simulink model "simulin"  (R2025b)
settings: Solver=VariableStepAuto  StartTime=0.0  StopTime=10.0  RelTol=1e-3
settings Model: Creator=viktor  LastModifiedBy=viktor

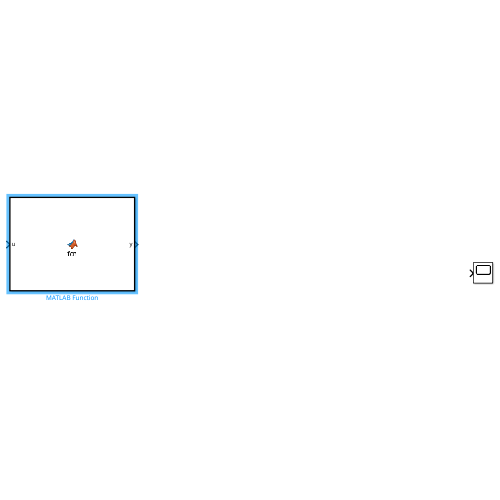
[thumbnail: Simulink's stored preview of the top-level diagram]
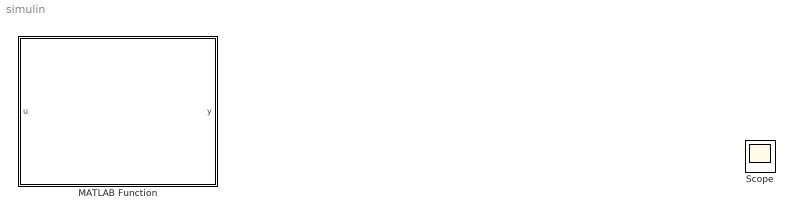
== system simulin ==
  MATLAB Function : MATLAB Function  TreatAsAtomicUnit=on
  Scope : Scope

== matlab function simulin/MATLAB Function ==
  data: u input; y output
function y = fcn(u)

y = u;
